simulink model "TwoLevelConverterIdealExample_Pejovic"  (R2023b)
settings: Solver=FixedStepDiscrete  StartTime=0.0  StopTime=100/fsw  MaxStep=1e-4  RelTol=1e-6  AbsTol=1e-6
PreLoadFcn:
  | ts = 1e-5; % local solver sample period
  | fsw = 1e3; % switching frequency
undefined symbols (not defined in the file): DiscIntNeverNeededParam, subcycleFactor
libraries: nesl_utility x53, fl_lib x52, ee_lib x16, simulink x12, fpga_utils_lib x12, eePwmGeneratorTwoLevel x1
(part 2 of 2)

== system TwoLevelConverterIdealExample_Pejovic/Inverter/Pejovic w//SCA/Switch6 ==
  G : Inport
  Controller : Subsystem  mask{threshold=threshold, Gs=Gs, s=timeScaling, avgFactor=avgFactor}
      mask prompts: Gs "Conductance (1/Ohm)"; s "Time scaling"; avgFactor "Subcycle average factor"
      mask DialogControl DescGroupVar Prompt: Description
      mask DialogControl Details Prompt: Switch Controller
  Gs : fl_lib/Electrical/Electrical Elements/Resistor  R=1/Gs Ohm  i_specify=off  i_priority=None  i=0 A  i_nominal_specify=off  i_nominal_unit=A  i_nominal_value=1  v_specify=off  v_priority=None  v=0 V  v_nominal_specify=off  v_nominal_unit=V  v_nominal_value=1
      settings: LibrarySourceBlock=SimscapeFPGAHIL_lib/Linearized Switch Models/Switch/Gs
  ic : fl_lib/Electrical/Electrical Sources/Controlled Current Source
      settings: LibrarySourceBlock=SimscapeFPGAHIL_lib/Linearized Switch Models/Switch/ic
  ic_in : nesl_utility/Simulink-PS Converter  PhysicalDomain=network_engine_domain  SubClassName=ps_input  LeftPortType=input  RightPortType=output  PseudoPeriodic=off  Frequencies=[]  NoiseDistribution=none  NoiseParameters=[]  Unit=A  AffineConversion=off  FilteringAndDerivatives=provide  SimscapeFilterOrder=1  InputFilterTimeConstant=0.001  UdotUserProvided=0
      settings: LibrarySourceBlock=SimscapeFPGAHIL_lib/Linearized Switch Models/Switch/ic_in
  is : fl_lib/Electrical/Electrical Sensors/Current Sensor
      settings: LibrarySourceBlock=SimscapeFPGAHIL_lib/Linearized Switch Models/Switch/is
  is_out : nesl_utility/PS-Simulink Converter  PhysicalDomain=network_engine_domain  SubClassName=ps_output  LeftPortType=input  RightPortType=output  PseudoPeriodic=off  Frequencies=[]  VectorFormat=1-D array  Unit=A  AffineConversion=off
      settings: LibrarySourceBlock=SimscapeFPGAHIL_lib/Linearized Switch Models/Switch/is_out
  vs : fl_lib/Electrical/Electrical Sensors/Voltage Sensor
      settings: LibrarySourceBlock=SimscapeFPGAHIL_lib/Linearized Switch Models/Switch/vs
  vs_out : nesl_utility/PS-Simulink Converter  PhysicalDomain=network_engine_domain  SubClassName=ps_output  LeftPortType=input  RightPortType=output  PseudoPeriodic=off  Frequencies=[]  VectorFormat=1-D array  Unit=V  AffineConversion=off
      settings: LibrarySourceBlock=SimscapeFPGAHIL_lib/Linearized Switch Models/Switch/vs_out
  + : PMIOPort  Side=Left
  - : PMIOPort  Port=2  Side=Right
  wires:
  vs_out/1 -> Controller/1(vs)
  is_out/1 -> Controller/2(is)
  G/1 -> Controller/3(G)
  Controller/1(ic) -> ic_in/1
  connections:
  ic/LConn1 -- Gs/LConn1 -- is/RConn2
  vs/RConn2 -- -/RConn1 -- Gs/RConn1 -- ic/RConn2
  vs/LConn1 -- +/RConn1 -- is/LConn1
  ic_in/RConn1 -- ic/RConn1
  vs_out/LConn1 -- vs/RConn1
  is_out/LConn1 -- is/RConn1

== system TwoLevelConverterIdealExample_Pejovic/Inverter/Simscape Converter/Gates ==
  Gates Simulink : Inport
  Demux : Demux  Outputs=6
  GaH : nesl_utility/Simulink-PS Converter  PhysicalDomain=network_engine_domain  SubClassName=ps_input  LeftPortType=input  RightPortType=output  PseudoPeriodic=off  Frequencies=[]  NoiseDistribution=none  NoiseParameters=[]  Unit=1  AffineConversion=off  FilteringAndDerivatives=zero  SimscapeFilterOrder=1  InputFilterTimeConstant=0.001  UdotUserProvided=0
  GaL : nesl_utility/Simulink-PS Converter  PhysicalDomain=network_engine_domain  SubClassName=ps_input  LeftPortType=input  RightPortType=output  PseudoPeriodic=off  Frequencies=[]  NoiseDistribution=none  NoiseParameters=[]  Unit=1  AffineConversion=off  FilteringAndDerivatives=zero  SimscapeFilterOrder=1  InputFilterTimeConstant=0.001  UdotUserProvided=0
  GbH : nesl_utility/Simulink-PS Converter  PhysicalDomain=network_engine_domain  SubClassName=ps_input  LeftPortType=input  RightPortType=output  PseudoPeriodic=off  Frequencies=[]  NoiseDistribution=none  NoiseParameters=[]  Unit=1  AffineConversion=off  FilteringAndDerivatives=zero  SimscapeFilterOrder=1  InputFilterTimeConstant=0.001  UdotUserProvided=0
  GbL : nesl_utility/Simulink-PS Converter  PhysicalDomain=network_engine_domain  SubClassName=ps_input  LeftPortType=input  RightPortType=output  PseudoPeriodic=off  Frequencies=[]  NoiseDistribution=none  NoiseParameters=[]  Unit=1  AffineConversion=off  FilteringAndDerivatives=zero  SimscapeFilterOrder=1  InputFilterTimeConstant=0.001  UdotUserProvided=0
  GcH : nesl_utility/Simulink-PS Converter  PhysicalDomain=network_engine_domain  SubClassName=ps_input  LeftPortType=input  RightPortType=output  PseudoPeriodic=off  Frequencies=[]  NoiseDistribution=none  NoiseParameters=[]  Unit=1  AffineConversion=off  FilteringAndDerivatives=zero  SimscapeFilterOrder=1  InputFilterTimeConstant=0.001  UdotUserProvided=0
  GcL : nesl_utility/Simulink-PS Converter  PhysicalDomain=network_engine_domain  SubClassName=ps_input  LeftPortType=input  RightPortType=output  PseudoPeriodic=off  Frequencies=[]  NoiseDistribution=none  NoiseParameters=[]  Unit=1  AffineConversion=off  FilteringAndDerivatives=zero  SimscapeFilterOrder=1  InputFilterTimeConstant=0.001  UdotUserProvided=0
  Six-Pulse Gate Multiplexer : ee_lib/Semiconductors & Converters/Converters/Six-Pulse Gate Multiplexer  port_option=ee.enum.controlport.ps
  Gates PS : PMIOPort  Side=Right
  wires:
  Demux/6 -> GcL/1
  Demux/3 -> GbH/1
  Demux/1 -> GaH/1
  Demux/4 -> GbL/1
  Demux/2 -> GaL/1
  Gates Simulink/1 -> Demux/1
  Demux/5 -> GcH/1
  connections:
  Six-Pulse Gate Multiplexer/LConn4 -- GbL/RConn1
  Six-Pulse Gate Multiplexer/LConn5 -- GcH/RConn1
  GaL/RConn1 -- Six-Pulse Gate Multiplexer/LConn2
  GaH/RConn1 -- Six-Pulse Gate Multiplexer/LConn1
  Six-Pulse Gate Multiplexer/LConn6 -- GcL/RConn1
  Six-Pulse Gate Multiplexer/LConn3 -- GbH/RConn1
  Six-Pulse Gate Multiplexer/RConn1 -- Gates PS/RConn1

== system TwoLevelConverterIdealExample_Pejovic/Inverter/Pejovic/Switch1/Controller ==
  vs : Inport
  is : Inport  Port=2
  G : Inport  Port=3
  Discrete-Time Integrator : DiscreteIntegrator  IntegratorMethod=Accumulation: Forward Euler  SampleTime=-1  ICPrevOutput=DiscIntNeverNeededParam  ICPrevScaledInput=DiscIntNeverNeededParam
  Gain : Gain  Gain=1/s
  Gain3 : Gain  Gain=Gs
  Subtract : Sum  Inputs=+-
  Switch State : Subsystem  Variant=on  VariantControl=Choice
  Unary Minus : UnaryMinus
  ic : Outport
  wires:
  vs/1 -> Gain3/1
  Gain/1 -> Discrete-Time Integrator/1
  Subtract/1 -> Gain/1
  Discrete-Time Integrator/1 -> ic/1, Subtract/2  "ic"
  is/1 -> Unary Minus/1
  Unary Minus/1 -> Switch State/1(on)  "on"
  G/1 -> Switch State/2(G)
  Gain3/1 -> Switch State/3(off)
  Switch State/1(ic) -> Subtract/1

== system TwoLevelConverterIdealExample_Pejovic/Inverter/Pejovic/Switch2/Controller ==
  vs : Inport
  is : Inport  Port=2
  G : Inport  Port=3
  Discrete-Time Integrator : DiscreteIntegrator  IntegratorMethod=Accumulation: Forward Euler  SampleTime=-1  ICPrevOutput=DiscIntNeverNeededParam  ICPrevScaledInput=DiscIntNeverNeededParam
  Gain : Gain  Gain=1/s
  Gain3 : Gain  Gain=Gs
  Subtract : Sum  Inputs=+-
  Switch State : Subsystem  Variant=on  VariantControl=Choice
  Unary Minus : UnaryMinus
  ic : Outport
  wires:
  Switch State/1(ic) -> Subtract/1
  Gain3/1 -> Switch State/3(off)
  G/1 -> Switch State/2(G)
  Unary Minus/1 -> Switch State/1(on)  "on"
  is/1 -> Unary Minus/1
  Discrete-Time Integrator/1 -> Subtract/2, ic/1  "ic"
  Subtract/1 -> Gain/1
  Gain/1 -> Discrete-Time Integrator/1
  vs/1 -> Gain3/1

== system TwoLevelConverterIdealExample_Pejovic/Inverter/Pejovic/Switch3/Controller ==
  vs : Inport
  is : Inport  Port=2
  G : Inport  Port=3
  Discrete-Time Integrator : DiscreteIntegrator  IntegratorMethod=Accumulation: Forward Euler  SampleTime=-1  ICPrevOutput=DiscIntNeverNeededParam  ICPrevScaledInput=DiscIntNeverNeededParam
  Gain : Gain  Gain=1/s
  Gain3 : Gain  Gain=Gs
  Subtract : Sum  Inputs=+-
  Switch State : Subsystem  Variant=on  VariantControl=Choice
  Unary Minus : UnaryMinus
  ic : Outport
  wires:
  vs/1 -> Gain3/1
  Gain/1 -> Discrete-Time Integrator/1
  Subtract/1 -> Gain/1
  Discrete-Time Integrator/1 -> ic/1, Subtract/2  "ic"
  is/1 -> Unary Minus/1
  Unary Minus/1 -> Switch State/1(on)  "on"
  G/1 -> Switch State/2(G)
  Gain3/1 -> Switch State/3(off)
  Switch State/1(ic) -> Subtract/1

== system TwoLevelConverterIdealExample_Pejovic/Inverter/Pejovic/Switch4/Controller ==
  vs : Inport
  is : Inport  Port=2
  G : Inport  Port=3
  Discrete-Time Integrator : DiscreteIntegrator  IntegratorMethod=Accumulation: Forward Euler  SampleTime=-1  ICPrevOutput=DiscIntNeverNeededParam  ICPrevScaledInput=DiscIntNeverNeededParam
  Gain : Gain  Gain=1/s
  Gain3 : Gain  Gain=Gs
  Subtract : Sum  Inputs=+-
  Switch State : Subsystem  Variant=on  VariantControl=Choice
  Unary Minus : UnaryMinus
  ic : Outport
  wires:
  Switch State/1(ic) -> Subtract/1
  Gain3/1 -> Switch State/3(off)
  G/1 -> Switch State/2(G)
  Unary Minus/1 -> Switch State/1(on)  "on"
  is/1 -> Unary Minus/1
  Discrete-Time Integrator/1 -> Subtract/2, ic/1  "ic"
  Subtract/1 -> Gain/1
  Gain/1 -> Discrete-Time Integrator/1
  vs/1 -> Gain3/1

== system TwoLevelConverterIdealExample_Pejovic/Inverter/Pejovic/Switch5/Controller ==
  vs : Inport
  is : Inport  Port=2
  G : Inport  Port=3
  Discrete-Time Integrator : DiscreteIntegrator  IntegratorMethod=Accumulation: Forward Euler  SampleTime=-1  ICPrevOutput=DiscIntNeverNeededParam  ICPrevScaledInput=DiscIntNeverNeededParam
  Gain : Gain  Gain=1/s
  Gain3 : Gain  Gain=Gs
  Subtract : Sum  Inputs=+-
  Switch State : Subsystem  Variant=on  VariantControl=Choice
  Unary Minus : UnaryMinus
  ic : Outport
  wires:
  vs/1 -> Gain3/1
  Gain/1 -> Discrete-Time Integrator/1
  Subtract/1 -> Gain/1
  Discrete-Time Integrator/1 -> ic/1, Subtract/2  "ic"
  is/1 -> Unary Minus/1
  Unary Minus/1 -> Switch State/1(on)  "on"
  G/1 -> Switch State/2(G)
  Gain3/1 -> Switch State/3(off)
  Switch State/1(ic) -> Subtract/1

== system TwoLevelConverterIdealExample_Pejovic/Inverter/Pejovic/Switch6/Controller ==
  vs : Inport
  is : Inport  Port=2
  G : Inport  Port=3
  Discrete-Time Integrator : DiscreteIntegrator  IntegratorMethod=Accumulation: Forward Euler  SampleTime=-1  ICPrevOutput=DiscIntNeverNeededParam  ICPrevScaledInput=DiscIntNeverNeededParam
  Gain : Gain  Gain=1/s
  Gain3 : Gain  Gain=Gs
  Subtract : Sum  Inputs=+-
  Switch State : Subsystem  Variant=on  VariantControl=Choice
  Unary Minus : UnaryMinus
  ic : Outport
  wires:
  Switch State/1(ic) -> Subtract/1
  Gain3/1 -> Switch State/3(off)
  G/1 -> Switch State/2(G)
  Unary Minus/1 -> Switch State/1(on)  "on"
  is/1 -> Unary Minus/1
  Discrete-Time Integrator/1 -> Subtract/2, ic/1  "ic"
  Subtract/1 -> Gain/1
  Gain/1 -> Discrete-Time Integrator/1
  vs/1 -> Gain3/1

== system TwoLevelConverterIdealExample_Pejovic/Inverter/Pejovic w//SCA/Switch1/Controller ==
  vs : Inport
  is : Inport  Port=2
  G : Inport  Port=3
  Discrete-Time Integrator : DiscreteIntegrator  IntegratorMethod=Accumulation: Forward Euler  SampleTime=-1  ICPrevOutput=DiscIntNeverNeededParam  ICPrevScaledInput=DiscIntNeverNeededParam
  Gain : Gain  Gain=1/s
  Gain3 : Gain  Gain=Gs
  Subtract : Sum  Inputs=+-
  Switch State : Subsystem  Variant=on  VariantControl=Choice
  Unary Minus : UnaryMinus
  ic : Outport
  wires:
  Switch State/1(ic) -> Subtract/1
  Gain3/1 -> Switch State/3(off)
  G/1 -> Switch State/2(G)
  Unary Minus/1 -> Switch State/1(on)  "on"
  is/1 -> Unary Minus/1
  Discrete-Time Integrator/1 -> Subtract/2, ic/1  "ic"
  Subtract/1 -> Gain/1
  Gain/1 -> Discrete-Time Integrator/1
  vs/1 -> Gain3/1

== system TwoLevelConverterIdealExample_Pejovic/Inverter/Pejovic w//SCA/Switch2/Controller ==
  vs : Inport
  is : Inport  Port=2
  G : Inport  Port=3
  Discrete-Time Integrator : DiscreteIntegrator  IntegratorMethod=Accumulation: Forward Euler  SampleTime=-1  ICPrevOutput=DiscIntNeverNeededParam  ICPrevScaledInput=DiscIntNeverNeededParam
  Gain : Gain  Gain=1/s
  Gain3 : Gain  Gain=Gs
  Subtract : Sum  Inputs=+-
  Switch State : Subsystem  Variant=on  VariantControl=Choice
  Unary Minus : UnaryMinus
  ic : Outport
  wires:
  vs/1 -> Gain3/1
  Gain/1 -> Discrete-Time Integrator/1
  Subtract/1 -> Gain/1
  Discrete-Time Integrator/1 -> ic/1, Subtract/2  "ic"
  is/1 -> Unary Minus/1
  Unary Minus/1 -> Switch State/1(on)  "on"
  G/1 -> Switch State/2(G)
  Gain3/1 -> Switch State/3(off)
  Switch State/1(ic) -> Subtract/1

== system TwoLevelConverterIdealExample_Pejovic/Inverter/Pejovic w//SCA/Switch3/Controller ==
  vs : Inport
  is : Inport  Port=2
  G : Inport  Port=3
  Discrete-Time Integrator : DiscreteIntegrator  IntegratorMethod=Accumulation: Forward Euler  SampleTime=-1  ICPrevOutput=DiscIntNeverNeededParam  ICPrevScaledInput=DiscIntNeverNeededParam
  Gain : Gain  Gain=1/s
  Gain3 : Gain  Gain=Gs
  Subtract : Sum  Inputs=+-
  Switch State : Subsystem  Variant=on  VariantControl=Choice
  Unary Minus : UnaryMinus
  ic : Outport
  wires:
  Switch State/1(ic) -> Subtract/1
  Gain3/1 -> Switch State/3(off)
  G/1 -> Switch State/2(G)
  Unary Minus/1 -> Switch State/1(on)  "on"
  is/1 -> Unary Minus/1
  Discrete-Time Integrator/1 -> Subtract/2, ic/1  "ic"
  Subtract/1 -> Gain/1
  Gain/1 -> Discrete-Time Integrator/1
  vs/1 -> Gain3/1

== system TwoLevelConverterIdealExample_Pejovic/Inverter/Pejovic w//SCA/Switch4/Controller ==
  vs : Inport
  is : Inport  Port=2
  G : Inport  Port=3
  Discrete-Time Integrator : DiscreteIntegrator  IntegratorMethod=Accumulation: Forward Euler  SampleTime=-1  ICPrevOutput=DiscIntNeverNeededParam  ICPrevScaledInput=DiscIntNeverNeededParam
  Gain : Gain  Gain=1/s
  Gain3 : Gain  Gain=Gs
  Subtract : Sum  Inputs=+-
  Switch State : Subsystem  Variant=on  VariantControl=Choice
  Unary Minus : UnaryMinus
  ic : Outport
  wires:
  vs/1 -> Gain3/1
  Gain/1 -> Discrete-Time Integrator/1
  Subtract/1 -> Gain/1
  Discrete-Time Integrator/1 -> ic/1, Subtract/2  "ic"
  is/1 -> Unary Minus/1
  Unary Minus/1 -> Switch State/1(on)  "on"
  G/1 -> Switch State/2(G)
  Gain3/1 -> Switch State/3(off)
  Switch State/1(ic) -> Subtract/1

== system TwoLevelConverterIdealExample_Pejovic/Inverter/Pejovic w//SCA/Switch5/Controller ==
  vs : Inport
  is : Inport  Port=2
  G : Inport  Port=3
  Discrete-Time Integrator : DiscreteIntegrator  IntegratorMethod=Accumulation: Forward Euler  SampleTime=-1  ICPrevOutput=DiscIntNeverNeededParam  ICPrevScaledInput=DiscIntNeverNeededParam
  Gain : Gain  Gain=1/s
  Gain3 : Gain  Gain=Gs
  Subtract : Sum  Inputs=+-
  Switch State : Subsystem  Variant=on  VariantControl=Choice
  Unary Minus : UnaryMinus
  ic : Outport
  wires:
  Switch State/1(ic) -> Subtract/1
  Gain3/1 -> Switch State/3(off)
  G/1 -> Switch State/2(G)
  Unary Minus/1 -> Switch State/1(on)  "on"
  is/1 -> Unary Minus/1
  Discrete-Time Integrator/1 -> Subtract/2, ic/1  "ic"
  Subtract/1 -> Gain/1
  Gain/1 -> Discrete-Time Integrator/1
  vs/1 -> Gain3/1

== system TwoLevelConverterIdealExample_Pejovic/Inverter/Pejovic w//SCA/Switch6/Controller ==
  vs : Inport
  is : Inport  Port=2
  G : Inport  Port=3
  Discrete-Time Integrator : DiscreteIntegrator  IntegratorMethod=Accumulation: Forward Euler  SampleTime=-1  ICPrevOutput=DiscIntNeverNeededParam  ICPrevScaledInput=DiscIntNeverNeededParam
  Gain : Gain  Gain=1/s
  Gain3 : Gain  Gain=Gs
  Subtract : Sum  Inputs=+-
  Switch State : Subsystem  Variant=on  VariantControl=Choice
  Unary Minus : UnaryMinus
  ic : Outport
  wires:
  vs/1 -> Gain3/1
  Gain/1 -> Discrete-Time Integrator/1
  Subtract/1 -> Gain/1
  Discrete-Time Integrator/1 -> ic/1, Subtract/2  "ic"
  is/1 -> Unary Minus/1
  Unary Minus/1 -> Switch State/1(on)  "on"
  G/1 -> Switch State/2(G)
  Gain3/1 -> Switch State/3(off)
  Switch State/1(ic) -> Subtract/1

== system TwoLevelConverterIdealExample_Pejovic/Inverter/Pejovic/Switch1/Controller/Switch State ==
  on : Inport
  G : Inport  Port=2
  off : Inport  Port=3
  Subcycle Average : Subsystem  VariantControl=avgFactor > 1
  Switch : Subsystem  VariantControl=avgFactor == 1
  ic : Outport

== system TwoLevelConverterIdealExample_Pejovic/Inverter/Pejovic/Switch2/Controller/Switch State ==
  on : Inport
  G : Inport  Port=2
  off : Inport  Port=3
  Subcycle Average : Subsystem  VariantControl=avgFactor > 1
  Switch : Subsystem  VariantControl=avgFactor == 1
  ic : Outport

== system TwoLevelConverterIdealExample_Pejovic/Inverter/Pejovic/Switch3/Controller/Switch State ==
  on : Inport
  G : Inport  Port=2
  off : Inport  Port=3
  Subcycle Average : Subsystem  VariantControl=avgFactor > 1
  Switch : Subsystem  VariantControl=avgFactor == 1
  ic : Outport

== system TwoLevelConverterIdealExample_Pejovic/Inverter/Pejovic/Switch4/Controller/Switch State ==
  on : Inport
  G : Inport  Port=2
  off : Inport  Port=3
  Subcycle Average : Subsystem  VariantControl=avgFactor > 1
  Switch : Subsystem  VariantControl=avgFactor == 1
  ic : Outport

== system TwoLevelConverterIdealExample_Pejovic/Inverter/Pejovic/Switch5/Controller/Switch State ==
  on : Inport
  G : Inport  Port=2
  off : Inport  Port=3
  Subcycle Average : Subsystem  VariantControl=avgFactor > 1
  Switch : Subsystem  VariantControl=avgFactor == 1
  ic : Outport

== system TwoLevelConverterIdealExample_Pejovic/Inverter/Pejovic/Switch6/Controller/Switch State ==
  on : Inport
  G : Inport  Port=2
  off : Inport  Port=3
  Subcycle Average : Subsystem  VariantControl=avgFactor > 1
  Switch : Subsystem  VariantControl=avgFactor == 1
  ic : Outport

== system TwoLevelConverterIdealExample_Pejovic/Inverter/Pejovic w//SCA/Switch1/Controller/Switch State ==
  on : Inport
  G : Inport  Port=2
  off : Inport  Port=3
  Subcycle Average : Subsystem  VariantControl=avgFactor > 1
  Switch : Subsystem  VariantControl=avgFactor == 1
  ic : Outport

== system TwoLevelConverterIdealExample_Pejovic/Inverter/Pejovic w//SCA/Switch2/Controller/Switch State ==
  on : Inport
  G : Inport  Port=2
  off : Inport  Port=3
  Subcycle Average : Subsystem  VariantControl=avgFactor > 1
  Switch : Subsystem  VariantControl=avgFactor == 1
  ic : Outport

== system TwoLevelConverterIdealExample_Pejovic/Inverter/Pejovic w//SCA/Switch3/Controller/Switch State ==
  on : Inport
  G : Inport  Port=2
  off : Inport  Port=3
  Subcycle Average : Subsystem  VariantControl=avgFactor > 1
  Switch : Subsystem  VariantControl=avgFactor == 1
  ic : Outport

== system TwoLevelConverterIdealExample_Pejovic/Inverter/Pejovic w//SCA/Switch4/Controller/Switch State ==
  on : Inport
  G : Inport  Port=2
  off : Inport  Port=3
  Subcycle Average : Subsystem  VariantControl=avgFactor > 1
  Switch : Subsystem  VariantControl=avgFactor == 1
  ic : Outport

== system TwoLevelConverterIdealExample_Pejovic/Inverter/Pejovic w//SCA/Switch5/Controller/Switch State ==
  on : Inport
  G : Inport  Port=2
  off : Inport  Port=3
  Subcycle Average : Subsystem  VariantControl=avgFactor > 1
  Switch : Subsystem  VariantControl=avgFactor == 1
  ic : Outport

== system TwoLevelConverterIdealExample_Pejovic/Inverter/Pejovic w//SCA/Switch6/Controller/Switch State ==
  on : Inport
  G : Inport  Port=2
  off : Inport  Port=3
  Subcycle Average : Subsystem  VariantControl=avgFactor > 1
  Switch : Subsystem  VariantControl=avgFactor == 1
  ic : Outport

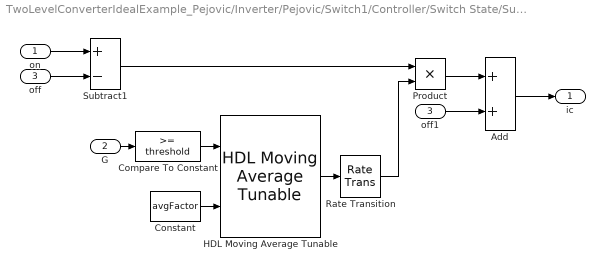
== system TwoLevelConverterIdealExample_Pejovic/Inverter/Pejovic/Switch1/Controller/Switch State/Subcycle Average ==
  on : Inport
  G : Inport  Port=2
  off : Inport  Port=3
  Add : Sum
  Compare To Constant : simulink/Logic and Bit Operations/Compare To Constant  relop=>=  const=threshold  OutDataTypeStr=boolean
  Constant : Constant  Value=avgFactor  OutDataTypeStr=uint16  SampleTime=-1
  HDL Moving Average Tunable : fpga_utils_lib/HDL Moving Average Tunable  SystemSampleTime=-1  VariantActivationTime=update diagram  AllowFlexibleInterface=on  Latency=0  AutoFrameSizeCalculation=off
  Product : Product  InputSameDT=on
  Rate Transition : RateTransition  OutPortSampleTimeOpt=Multiple of input port sample time  OutPortSampleTimeMultiple=avgFactor
  Subtract1 : Sum  Inputs=+-
  off1 : InportShadow  Port=3
  ic : Outport
  wires:
  on/1 -> Subtract1/1
  off/1 -> Subtract1/2
  Constant/1 -> HDL Moving Average Tunable/2
  HDL Moving Average Tunable/1 -> Rate Transition/1
  G/1 -> Compare To Constant/1
  Compare To Constant/1 -> HDL Moving Average Tunable/1
  Subtract1/1 -> Product/1
  Rate Transition/1 -> Product/2
  Product/1 -> Add/1
  Add/1 -> ic/1
  off1/1 -> Add/2

== system TwoLevelConverterIdealExample_Pejovic/Inverter/Pejovic/Switch1/Controller/Switch State/Switch ==
  on : Inport
  G : Inport  Port=2
  off : Inport  Port=3
  S2 : Switch  Threshold=threshold  SaturateOnIntegerOverflow=off  InputSameDT=off
  ic : Outport
  wires:
  on/1 -> S2/1
  S2/1 -> ic/1
  G/1 -> S2/2
  off/1 -> S2/3

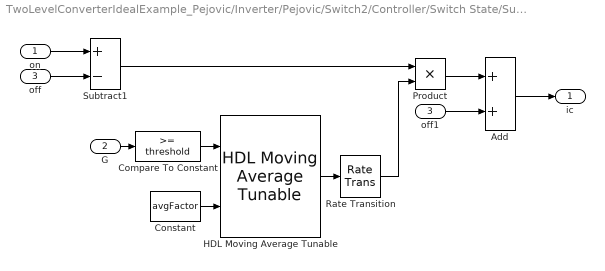
== system TwoLevelConverterIdealExample_Pejovic/Inverter/Pejovic/Switch2/Controller/Switch State/Subcycle Average ==
  on : Inport
  G : Inport  Port=2
  off : Inport  Port=3
  Add : Sum
  Compare To Constant : simulink/Logic and Bit Operations/Compare To Constant  relop=>=  const=threshold  OutDataTypeStr=boolean
  Constant : Constant  Value=avgFactor  OutDataTypeStr=uint16  SampleTime=-1
  HDL Moving Average Tunable : fpga_utils_lib/HDL Moving Average Tunable  SystemSampleTime=-1  VariantActivationTime=update diagram  AllowFlexibleInterface=on  Latency=0  AutoFrameSizeCalculation=off
  Product : Product  InputSameDT=on
  Rate Transition : RateTransition  OutPortSampleTimeOpt=Multiple of input port sample time  OutPortSampleTimeMultiple=avgFactor
  Subtract1 : Sum  Inputs=+-
  off1 : InportShadow  Port=3
  ic : Outport
  wires:
  off1/1 -> Add/2
  Add/1 -> ic/1
  Product/1 -> Add/1
  Rate Transition/1 -> Product/2
  Subtract1/1 -> Product/1
  Compare To Constant/1 -> HDL Moving Average Tunable/1
  G/1 -> Compare To Constant/1
  HDL Moving Average Tunable/1 -> Rate Transition/1
  Constant/1 -> HDL Moving Average Tunable/2
  off/1 -> Subtract1/2
  on/1 -> Subtract1/1

== system TwoLevelConverterIdealExample_Pejovic/Inverter/Pejovic/Switch2/Controller/Switch State/Switch ==
  on : Inport
  G : Inport  Port=2
  off : Inport  Port=3
  S2 : Switch  Threshold=threshold  SaturateOnIntegerOverflow=off  InputSameDT=off
  ic : Outport
  wires:
  off/1 -> S2/3
  G/1 -> S2/2
  S2/1 -> ic/1
  on/1 -> S2/1

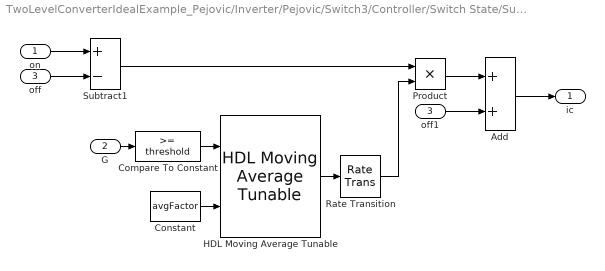
== system TwoLevelConverterIdealExample_Pejovic/Inverter/Pejovic/Switch3/Controller/Switch State/Subcycle Average ==
  on : Inport
  G : Inport  Port=2
  off : Inport  Port=3
  Add : Sum
  Compare To Constant : simulink/Logic and Bit Operations/Compare To Constant  relop=>=  const=threshold  OutDataTypeStr=boolean
  Constant : Constant  Value=avgFactor  OutDataTypeStr=uint16  SampleTime=-1
  HDL Moving Average Tunable : fpga_utils_lib/HDL Moving Average Tunable  SystemSampleTime=-1  VariantActivationTime=update diagram  AllowFlexibleInterface=on  Latency=0  AutoFrameSizeCalculation=off
  Product : Product  InputSameDT=on
  Rate Transition : RateTransition  OutPortSampleTimeOpt=Multiple of input port sample time  OutPortSampleTimeMultiple=avgFactor
  Subtract1 : Sum  Inputs=+-
  off1 : InportShadow  Port=3
  ic : Outport
  wires:
  on/1 -> Subtract1/1
  off/1 -> Subtract1/2
  Constant/1 -> HDL Moving Average Tunable/2
  HDL Moving Average Tunable/1 -> Rate Transition/1
  G/1 -> Compare To Constant/1
  Compare To Constant/1 -> HDL Moving Average Tunable/1
  Subtract1/1 -> Product/1
  Rate Transition/1 -> Product/2
  Product/1 -> Add/1
  Add/1 -> ic/1
  off1/1 -> Add/2

== system TwoLevelConverterIdealExample_Pejovic/Inverter/Pejovic/Switch3/Controller/Switch State/Switch ==
  on : Inport
  G : Inport  Port=2
  off : Inport  Port=3
  S2 : Switch  Threshold=threshold  SaturateOnIntegerOverflow=off  InputSameDT=off
  ic : Outport
  wires:
  on/1 -> S2/1
  S2/1 -> ic/1
  G/1 -> S2/2
  off/1 -> S2/3

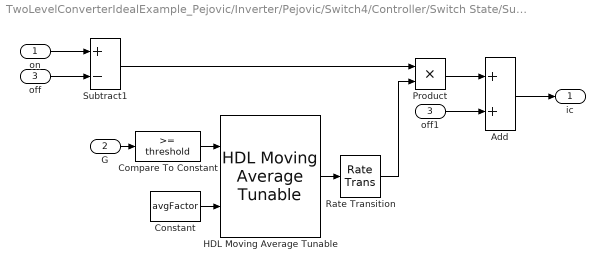
== system TwoLevelConverterIdealExample_Pejovic/Inverter/Pejovic/Switch4/Controller/Switch State/Subcycle Average ==
  on : Inport
  G : Inport  Port=2
  off : Inport  Port=3
  Add : Sum
  Compare To Constant : simulink/Logic and Bit Operations/Compare To Constant  relop=>=  const=threshold  OutDataTypeStr=boolean
  Constant : Constant  Value=avgFactor  OutDataTypeStr=uint16  SampleTime=-1
  HDL Moving Average Tunable : fpga_utils_lib/HDL Moving Average Tunable  SystemSampleTime=-1  VariantActivationTime=update diagram  AllowFlexibleInterface=on  Latency=0  AutoFrameSizeCalculation=off
  Product : Product  InputSameDT=on
  Rate Transition : RateTransition  OutPortSampleTimeOpt=Multiple of input port sample time  OutPortSampleTimeMultiple=avgFactor
  Subtract1 : Sum  Inputs=+-
  off1 : InportShadow  Port=3
  ic : Outport
  wires:
  off1/1 -> Add/2
  Add/1 -> ic/1
  Product/1 -> Add/1
  Rate Transition/1 -> Product/2
  Subtract1/1 -> Product/1
  Compare To Constant/1 -> HDL Moving Average Tunable/1
  G/1 -> Compare To Constant/1
  HDL Moving Average Tunable/1 -> Rate Transition/1
  Constant/1 -> HDL Moving Average Tunable/2
  off/1 -> Subtract1/2
  on/1 -> Subtract1/1

== system TwoLevelConverterIdealExample_Pejovic/Inverter/Pejovic/Switch4/Controller/Switch State/Switch ==
  on : Inport
  G : Inport  Port=2
  off : Inport  Port=3
  S2 : Switch  Threshold=threshold  SaturateOnIntegerOverflow=off  InputSameDT=off
  ic : Outport
  wires:
  off/1 -> S2/3
  G/1 -> S2/2
  S2/1 -> ic/1
  on/1 -> S2/1

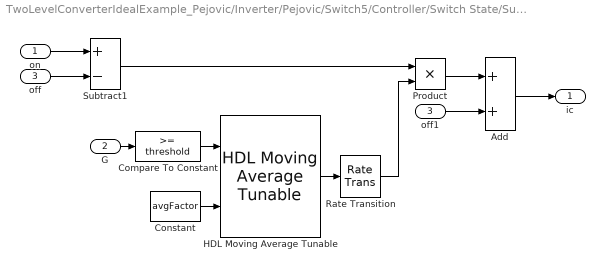
== system TwoLevelConverterIdealExample_Pejovic/Inverter/Pejovic/Switch5/Controller/Switch State/Subcycle Average ==
  on : Inport
  G : Inport  Port=2
  off : Inport  Port=3
  Add : Sum
  Compare To Constant : simulink/Logic and Bit Operations/Compare To Constant  relop=>=  const=threshold  OutDataTypeStr=boolean
  Constant : Constant  Value=avgFactor  OutDataTypeStr=uint16  SampleTime=-1
  HDL Moving Average Tunable : fpga_utils_lib/HDL Moving Average Tunable  SystemSampleTime=-1  VariantActivationTime=update diagram  AllowFlexibleInterface=on  Latency=0  AutoFrameSizeCalculation=off
  Product : Product  InputSameDT=on
  Rate Transition : RateTransition  OutPortSampleTimeOpt=Multiple of input port sample time  OutPortSampleTimeMultiple=avgFactor
  Subtract1 : Sum  Inputs=+-
  off1 : InportShadow  Port=3
  ic : Outport
  wires:
  on/1 -> Subtract1/1
  off/1 -> Subtract1/2
  Constant/1 -> HDL Moving Average Tunable/2
  HDL Moving Average Tunable/1 -> Rate Transition/1
  G/1 -> Compare To Constant/1
  Compare To Constant/1 -> HDL Moving Average Tunable/1
  Subtract1/1 -> Product/1
  Rate Transition/1 -> Product/2
  Product/1 -> Add/1
  Add/1 -> ic/1
  off1/1 -> Add/2

== system TwoLevelConverterIdealExample_Pejovic/Inverter/Pejovic/Switch5/Controller/Switch State/Switch ==
  on : Inport
  G : Inport  Port=2
  off : Inport  Port=3
  S2 : Switch  Threshold=threshold  SaturateOnIntegerOverflow=off  InputSameDT=off
  ic : Outport
  wires:
  on/1 -> S2/1
  S2/1 -> ic/1
  G/1 -> S2/2
  off/1 -> S2/3

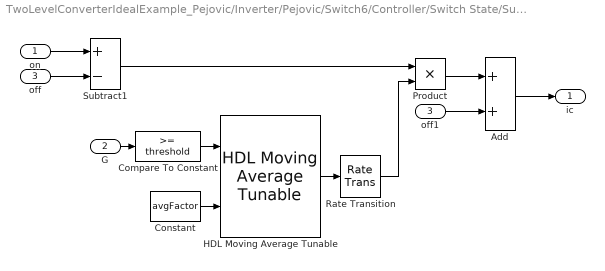
== system TwoLevelConverterIdealExample_Pejovic/Inverter/Pejovic/Switch6/Controller/Switch State/Subcycle Average ==
  on : Inport
  G : Inport  Port=2
  off : Inport  Port=3
  Add : Sum
  Compare To Constant : simulink/Logic and Bit Operations/Compare To Constant  relop=>=  const=threshold  OutDataTypeStr=boolean
  Constant : Constant  Value=avgFactor  OutDataTypeStr=uint16  SampleTime=-1
  HDL Moving Average Tunable : fpga_utils_lib/HDL Moving Average Tunable  SystemSampleTime=-1  VariantActivationTime=update diagram  AllowFlexibleInterface=on  Latency=0  AutoFrameSizeCalculation=off
  Product : Product  InputSameDT=on
  Rate Transition : RateTransition  OutPortSampleTimeOpt=Multiple of input port sample time  OutPortSampleTimeMultiple=avgFactor
  Subtract1 : Sum  Inputs=+-
  off1 : InportShadow  Port=3
  ic : Outport
  wires:
  off1/1 -> Add/2
  Add/1 -> ic/1
  Product/1 -> Add/1
  Rate Transition/1 -> Product/2
  Subtract1/1 -> Product/1
  Compare To Constant/1 -> HDL Moving Average Tunable/1
  G/1 -> Compare To Constant/1
  HDL Moving Average Tunable/1 -> Rate Transition/1
  Constant/1 -> HDL Moving Average Tunable/2
  off/1 -> Subtract1/2
  on/1 -> Subtract1/1

== system TwoLevelConverterIdealExample_Pejovic/Inverter/Pejovic/Switch6/Controller/Switch State/Switch ==
  on : Inport
  G : Inport  Port=2
  off : Inport  Port=3
  S2 : Switch  Threshold=threshold  SaturateOnIntegerOverflow=off  InputSameDT=off
  ic : Outport
  wires:
  off/1 -> S2/3
  G/1 -> S2/2
  S2/1 -> ic/1
  on/1 -> S2/1

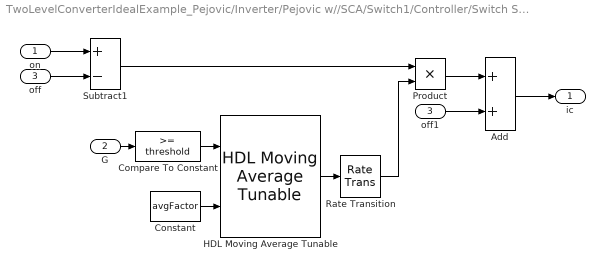
== system TwoLevelConverterIdealExample_Pejovic/Inverter/Pejovic w//SCA/Switch1/Controller/Switch State/Subcycle Average ==
  on : Inport
  G : Inport  Port=2
  off : Inport  Port=3
  Add : Sum
  Compare To Constant : simulink/Logic and Bit Operations/Compare To Constant  relop=>=  const=threshold  OutDataTypeStr=boolean
  Constant : Constant  Value=avgFactor  OutDataTypeStr=uint16  SampleTime=-1
  HDL Moving Average Tunable : fpga_utils_lib/HDL Moving Average Tunable  SystemSampleTime=-1  VariantActivationTime=update diagram  AllowFlexibleInterface=on  Latency=0  AutoFrameSizeCalculation=off
  Product : Product  InputSameDT=on
  Rate Transition : RateTransition  OutPortSampleTimeOpt=Multiple of input port sample time  OutPortSampleTimeMultiple=avgFactor
  Subtract1 : Sum  Inputs=+-
  off1 : InportShadow  Port=3
  ic : Outport
  wires:
  off1/1 -> Add/2
  Add/1 -> ic/1
  Product/1 -> Add/1
  Rate Transition/1 -> Product/2
  Subtract1/1 -> Product/1
  Compare To Constant/1 -> HDL Moving Average Tunable/1
  G/1 -> Compare To Constant/1
  HDL Moving Average Tunable/1 -> Rate Transition/1
  Constant/1 -> HDL Moving Average Tunable/2
  off/1 -> Subtract1/2
  on/1 -> Subtract1/1

== system TwoLevelConverterIdealExample_Pejovic/Inverter/Pejovic w//SCA/Switch1/Controller/Switch State/Switch ==
  on : Inport
  G : Inport  Port=2
  off : Inport  Port=3
  S2 : Switch  Threshold=threshold  SaturateOnIntegerOverflow=off  InputSameDT=off
  ic : Outport
  wires:
  off/1 -> S2/3
  G/1 -> S2/2
  S2/1 -> ic/1
  on/1 -> S2/1

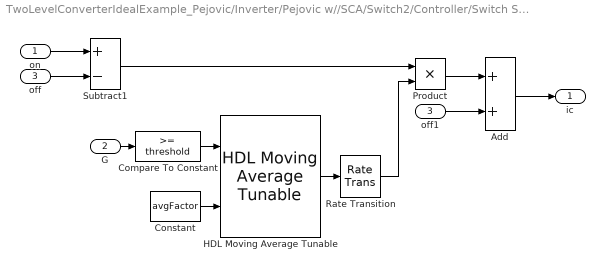
== system TwoLevelConverterIdealExample_Pejovic/Inverter/Pejovic w//SCA/Switch2/Controller/Switch State/Subcycle Average ==
  on : Inport
  G : Inport  Port=2
  off : Inport  Port=3
  Add : Sum
  Compare To Constant : simulink/Logic and Bit Operations/Compare To Constant  relop=>=  const=threshold  OutDataTypeStr=boolean
  Constant : Constant  Value=avgFactor  OutDataTypeStr=uint16  SampleTime=-1
  HDL Moving Average Tunable : fpga_utils_lib/HDL Moving Average Tunable  SystemSampleTime=-1  VariantActivationTime=update diagram  AllowFlexibleInterface=on  Latency=0  AutoFrameSizeCalculation=off
  Product : Product  InputSameDT=on
  Rate Transition : RateTransition  OutPortSampleTimeOpt=Multiple of input port sample time  OutPortSampleTimeMultiple=avgFactor
  Subtract1 : Sum  Inputs=+-
  off1 : InportShadow  Port=3
  ic : Outport
  wires:
  on/1 -> Subtract1/1
  off/1 -> Subtract1/2
  Constant/1 -> HDL Moving Average Tunable/2
  HDL Moving Average Tunable/1 -> Rate Transition/1
  G/1 -> Compare To Constant/1
  Compare To Constant/1 -> HDL Moving Average Tunable/1
  Subtract1/1 -> Product/1
  Rate Transition/1 -> Product/2
  Product/1 -> Add/1
  Add/1 -> ic/1
  off1/1 -> Add/2

== system TwoLevelConverterIdealExample_Pejovic/Inverter/Pejovic w//SCA/Switch2/Controller/Switch State/Switch ==
  on : Inport
  G : Inport  Port=2
  off : Inport  Port=3
  S2 : Switch  Threshold=threshold  SaturateOnIntegerOverflow=off  InputSameDT=off
  ic : Outport
  wires:
  on/1 -> S2/1
  S2/1 -> ic/1
  G/1 -> S2/2
  off/1 -> S2/3

== system TwoLevelConverterIdealExample_Pejovic/Inverter/Pejovic w//SCA/Switch3/Controller/Switch State/Subcycle Average ==
  on : Inport
  G : Inport  Port=2
  off : Inport  Port=3
  Add : Sum
  Compare To Constant : simulink/Logic and Bit Operations/Compare To Constant  relop=>=  const=threshold  OutDataTypeStr=boolean
  Constant : Constant  Value=avgFactor  OutDataTypeStr=uint16  SampleTime=-1
  HDL Moving Average Tunable : fpga_utils_lib/HDL Moving Average Tunable  SystemSampleTime=-1  VariantActivationTime=update diagram  AllowFlexibleInterface=on  Latency=0  AutoFrameSizeCalculation=off
  Product : Product  InputSameDT=on
  Rate Transition : RateTransition  OutPortSampleTimeOpt=Multiple of input port sample time  OutPortSampleTimeMultiple=avgFactor
  Subtract1 : Sum  Inputs=+-
  off1 : InportShadow  Port=3
  ic : Outport
  wires:
  off1/1 -> Add/2
  Add/1 -> ic/1
  Product/1 -> Add/1
  Rate Transition/1 -> Product/2
  Subtract1/1 -> Product/1
  Compare To Constant/1 -> HDL Moving Average Tunable/1
  G/1 -> Compare To Constant/1
  HDL Moving Average Tunable/1 -> Rate Transition/1
  Constant/1 -> HDL Moving Average Tunable/2
  off/1 -> Subtract1/2
  on/1 -> Subtract1/1

== system TwoLevelConverterIdealExample_Pejovic/Inverter/Pejovic w//SCA/Switch3/Controller/Switch State/Switch ==
  on : Inport
  G : Inport  Port=2
  off : Inport  Port=3
  S2 : Switch  Threshold=threshold  SaturateOnIntegerOverflow=off  InputSameDT=off
  ic : Outport
  wires:
  off/1 -> S2/3
  G/1 -> S2/2
  S2/1 -> ic/1
  on/1 -> S2/1

== system TwoLevelConverterIdealExample_Pejovic/Inverter/Pejovic w//SCA/Switch4/Controller/Switch State/Subcycle Average ==
  on : Inport
  G : Inport  Port=2
  off : Inport  Port=3
  Add : Sum
  Compare To Constant : simulink/Logic and Bit Operations/Compare To Constant  relop=>=  const=threshold  OutDataTypeStr=boolean
  Constant : Constant  Value=avgFactor  OutDataTypeStr=uint16  SampleTime=-1
  HDL Moving Average Tunable : fpga_utils_lib/HDL Moving Average Tunable  SystemSampleTime=-1  VariantActivationTime=update diagram  AllowFlexibleInterface=on  Latency=0  AutoFrameSizeCalculation=off
  Product : Product  InputSameDT=on
  Rate Transition : RateTransition  OutPortSampleTimeOpt=Multiple of input port sample time  OutPortSampleTimeMultiple=avgFactor
  Subtract1 : Sum  Inputs=+-
  off1 : InportShadow  Port=3
  ic : Outport
  wires:
  on/1 -> Subtract1/1
  off/1 -> Subtract1/2
  Constant/1 -> HDL Moving Average Tunable/2
  HDL Moving Average Tunable/1 -> Rate Transition/1
  G/1 -> Compare To Constant/1
  Compare To Constant/1 -> HDL Moving Average Tunable/1
  Subtract1/1 -> Product/1
  Rate Transition/1 -> Product/2
  Product/1 -> Add/1
  Add/1 -> ic/1
  off1/1 -> Add/2

== system TwoLevelConverterIdealExample_Pejovic/Inverter/Pejovic w//SCA/Switch4/Controller/Switch State/Switch ==
  on : Inport
  G : Inport  Port=2
  off : Inport  Port=3
  S2 : Switch  Threshold=threshold  SaturateOnIntegerOverflow=off  InputSameDT=off
  ic : Outport
  wires:
  on/1 -> S2/1
  S2/1 -> ic/1
  G/1 -> S2/2
  off/1 -> S2/3

== system TwoLevelConverterIdealExample_Pejovic/Inverter/Pejovic w//SCA/Switch5/Controller/Switch State/Subcycle Average ==
  on : Inport
  G : Inport  Port=2
  off : Inport  Port=3
  Add : Sum
  Compare To Constant : simulink/Logic and Bit Operations/Compare To Constant  relop=>=  const=threshold  OutDataTypeStr=boolean
  Constant : Constant  Value=avgFactor  OutDataTypeStr=uint16  SampleTime=-1
  HDL Moving Average Tunable : fpga_utils_lib/HDL Moving Average Tunable  SystemSampleTime=-1  VariantActivationTime=update diagram  AllowFlexibleInterface=on  Latency=0  AutoFrameSizeCalculation=off
  Product : Product  InputSameDT=on
  Rate Transition : RateTransition  OutPortSampleTimeOpt=Multiple of input port sample time  OutPortSampleTimeMultiple=avgFactor
  Subtract1 : Sum  Inputs=+-
  off1 : InportShadow  Port=3
  ic : Outport
  wires:
  off1/1 -> Add/2
  Add/1 -> ic/1
  Product/1 -> Add/1
  Rate Transition/1 -> Product/2
  Subtract1/1 -> Product/1
  Compare To Constant/1 -> HDL Moving Average Tunable/1
  G/1 -> Compare To Constant/1
  HDL Moving Average Tunable/1 -> Rate Transition/1
  Constant/1 -> HDL Moving Average Tunable/2
  off/1 -> Subtract1/2
  on/1 -> Subtract1/1

== system TwoLevelConverterIdealExample_Pejovic/Inverter/Pejovic w//SCA/Switch5/Controller/Switch State/Switch ==
  on : Inport
  G : Inport  Port=2
  off : Inport  Port=3
  S2 : Switch  Threshold=threshold  SaturateOnIntegerOverflow=off  InputSameDT=off
  ic : Outport
  wires:
  off/1 -> S2/3
  G/1 -> S2/2
  S2/1 -> ic/1
  on/1 -> S2/1

== system TwoLevelConverterIdealExample_Pejovic/Inverter/Pejovic w//SCA/Switch6/Controller/Switch State/Subcycle Average ==
  on : Inport
  G : Inport  Port=2
  off : Inport  Port=3
  Add : Sum
  Compare To Constant : simulink/Logic and Bit Operations/Compare To Constant  relop=>=  const=threshold  OutDataTypeStr=boolean
  Constant : Constant  Value=avgFactor  OutDataTypeStr=uint16  SampleTime=-1
  HDL Moving Average Tunable : fpga_utils_lib/HDL Moving Average Tunable  SystemSampleTime=-1  VariantActivationTime=update diagram  AllowFlexibleInterface=on  Latency=0  AutoFrameSizeCalculation=off
  Product : Product  InputSameDT=on
  Rate Transition : RateTransition  OutPortSampleTimeOpt=Multiple of input port sample time  OutPortSampleTimeMultiple=avgFactor
  Subtract1 : Sum  Inputs=+-
  off1 : InportShadow  Port=3
  ic : Outport
  wires:
  on/1 -> Subtract1/1
  off/1 -> Subtract1/2
  Constant/1 -> HDL Moving Average Tunable/2
  HDL Moving Average Tunable/1 -> Rate Transition/1
  G/1 -> Compare To Constant/1
  Compare To Constant/1 -> HDL Moving Average Tunable/1
  Subtract1/1 -> Product/1
  Rate Transition/1 -> Product/2
  Product/1 -> Add/1
  Add/1 -> ic/1
  off1/1 -> Add/2

== system TwoLevelConverterIdealExample_Pejovic/Inverter/Pejovic w//SCA/Switch6/Controller/Switch State/Switch ==
  on : Inport
  G : Inport  Port=2
  off : Inport  Port=3
  S2 : Switch  Threshold=threshold  SaturateOnIntegerOverflow=off  InputSameDT=off
  ic : Outport
  wires:
  on/1 -> S2/1
  S2/1 -> ic/1
  G/1 -> S2/2
  off/1 -> S2/3
